simulink model "model_perturb_input"  (R2023b)
settings: Solver=VariableStepAuto  StartTime=0.0  StopTime=0.03  RelTol=1e-3
values from neighbouring files (symbols this model uses):
  A = 8    [project.m]    (also in projectAB.m)
  C = 0.176    [project.m]    (also in projectAB.m = C_2)
  denPI = denPI{1,1}    [projectAB.m]
  kp = 9.34    [projectAB.m]
  kr = 0.2    [projectAB.m]
  ku = 0.5    [project.m]    (also in projectAB.m = 0.65)
  L2 = L*10    [projectAB.m]
  numPI = numPI{1,1}    [projectAB.m]
  Rs = 2.4    [project.m]    (also in projectAB.m)
  U2 = 12    [project.m]    (also in projectAB.m)
  Udc = ku*sqrt(2)*U2    [projectAB.m]
settings Model: Creator=pierpatrat  LastModifiedBy=pierpatrat

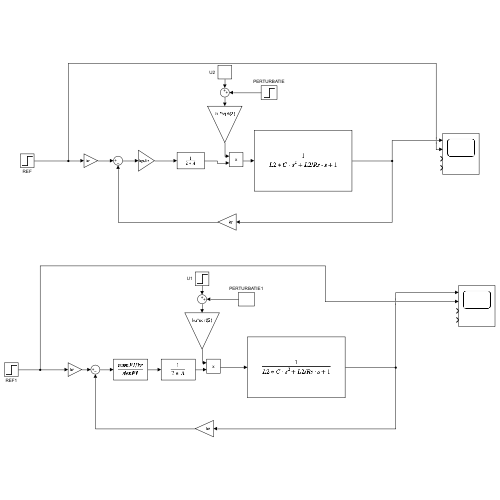
[thumbnail: Simulink's stored preview of the top-level diagram]
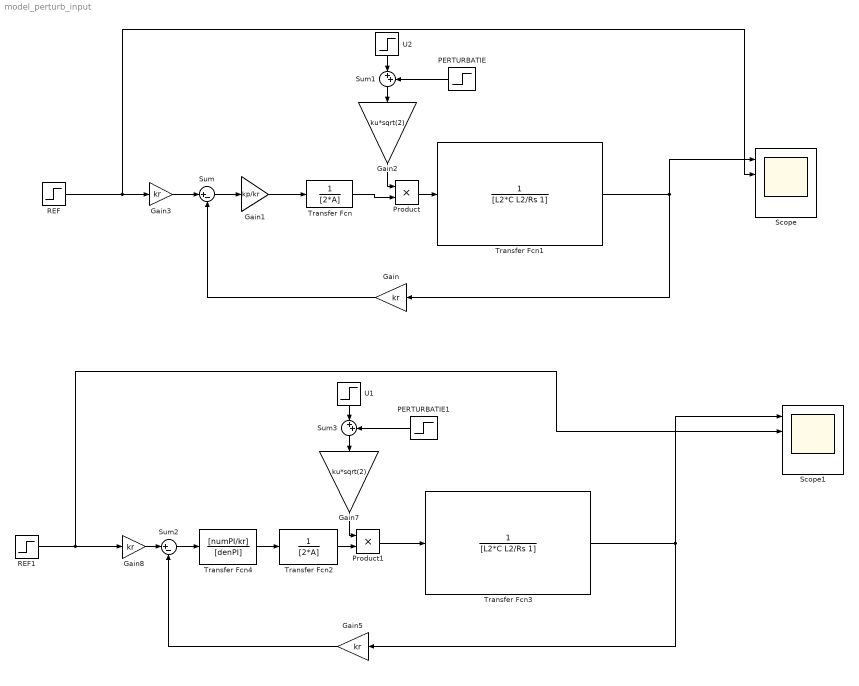
== system model_perturb_input ==
  Gain{,3,5,8} (4 alike) : Gain  Gain=kr
  Gain1 : Gain  Gain=kp/kr
  Gain2 : Gain  Gain=ku*sqrt(2)
  Gain7 : Gain  Gain=ku*sqrt(2)
  PERTURBATIE : Step  Time=0.005  After=0.1*U2  SampleTime=0
  PERTURBATIE1 : Step  Time=0.005  After=0.1*U2  SampleTime=0
  Product : Product
  Product1 : Product
  REF : Step  Time=0  After=Udc  SampleTime=0.0000001
  REF1 : Step  Time=0  After=Udc  SampleTime=0.0000001
  Scope : Scope  NumInputPorts=4
  Scope1 : Scope  NumInputPorts=4
  Sum : Sum  Inputs=|+-
  Sum1 : Sum  Inputs=|++
  Sum2 : Sum  Inputs=|+-
  Sum3 : Sum  Inputs=|++
  Transfer Fcn : TransferFcn  Denominator=[2*A]
  Transfer Fcn1 : TransferFcn  Denominator=[L2*C L2/Rs 1]
  Transfer Fcn2 : TransferFcn  Denominator=[2*A]
  Transfer Fcn3 : TransferFcn  Denominator=[L2*C L2/Rs 1]
  Transfer Fcn4 : TransferFcn  Numerator=[numPI/kr]  Denominator=[denPI]
  U1 : Step  Time=0  After=U2  SampleTime=0
  U2 : Step  Time=0  After=U2  SampleTime=0
  wires:
  Product/1 -> Transfer Fcn1/1
  Gain/1 -> Sum/2
  Transfer Fcn1/1 -> Gain/1, Scope/1
  Sum/1 -> Gain1/1
  Gain1/1 -> Transfer Fcn/1
  Transfer Fcn/1 -> Product/2
  Gain3/1 -> Sum/1
  REF/1 -> Gain3/1, Scope/2
  Gain2/1 -> Product/1
  U2/1 -> Sum1/1
  Sum1/1 -> Gain2/1
  PERTURBATIE/1 -> Sum1/2
  Transfer Fcn2/1 -> Product1/2
  Product1/1 -> Transfer Fcn3/1
  Sum3/1 -> Gain7/1
  U1/1 -> Sum3/1
  PERTURBATIE1/1 -> Sum3/2
  Gain7/1 -> Product1/1
  Gain5/1 -> Sum2/2
  REF1/1 -> Gain8/1, Scope1/2
  Transfer Fcn4/1 -> Transfer Fcn2/1
  Transfer Fcn3/1 -> Gain5/1, Scope1/1
  Gain8/1 -> Sum2/1
  Sum2/1 -> Transfer Fcn4/1
